simulink model "multiagent"  (R2018b)
settings: Solver=ode4  StartTime=0.0  StopTime=tmax  FixedStep=0.005  RelTol=1e-3
undefined symbols (not defined in the file): dq1_init, dq2_init, dq3_init, dq4_init, q1_init, q2_init, q3_init, q4_init
settings Model: Creator=q5461  LastModifiedBy=q5461

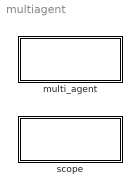
== system multiagent ==
  multi_agent : Subsystem
  scope : Subsystem

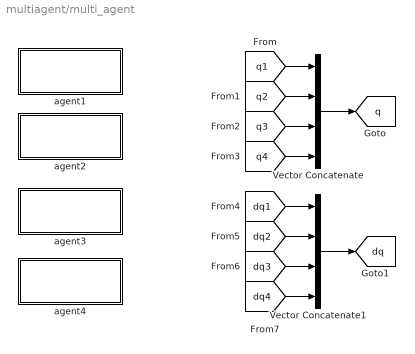
== system multiagent/multi_agent ==
  Vector Concatenate : Concatenate  NumInputs=4
  Vector Concatenate1 : Concatenate  NumInputs=4
  agent1 : Subsystem
  agent2 : Subsystem
  agent3 : Subsystem
  agent4 : Subsystem
  tag scope: dq=global, q=global
  wires:
  [q1] -> Vector Concatenate/1
  [q2] -> Vector Concatenate/2
  Vector Concatenate/1 -> [q]
  [q3] -> Vector Concatenate/3
  [q4] -> Vector Concatenate/4
  [dq4] -> Vector Concatenate1/4
  [dq3] -> Vector Concatenate1/3
  Vector Concatenate1/1 -> [dq]
  [dq2] -> Vector Concatenate1/2
  [dq1] -> Vector Concatenate1/1

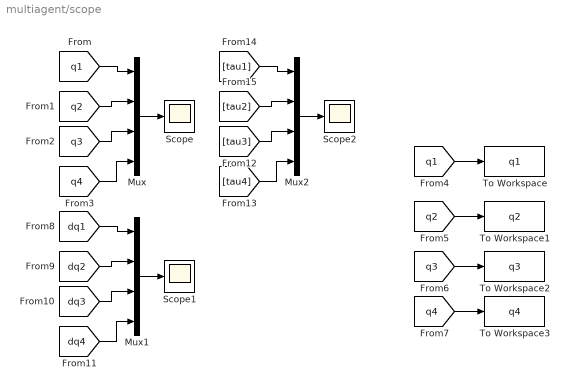
== system multiagent/scope ==
  Mux : Mux
  Mux1 : Mux
  Mux2 : Mux
  Scope : Scope
  Scope1 : Scope
  Scope2 : Scope
  To Workspace : ToWorkspace  VariableName=q1  SaveFormat=Timeseries  SampleTime=-1
  To Workspace1 : ToWorkspace  VariableName=q2  SaveFormat=Timeseries  SampleTime=-1
  To Workspace2 : ToWorkspace  VariableName=q3  SaveFormat=Timeseries  SampleTime=-1
  To Workspace3 : ToWorkspace  VariableName=q4  SaveFormat=Timeseries  SampleTime=-1
  wires:
  Mux/1 -> Scope/1
  [q1] -> Mux/1
  [q2] -> Mux/2
  [q3] -> Mux/3
  [q4] -> Mux/4
  [q1] -> To Workspace/1
  [q2] -> To Workspace1/1
  [q3] -> To Workspace2/1
  [q4] -> To Workspace3/1
  [dq4] -> Mux1/4
  [dq3] -> Mux1/3
  [dq2] -> Mux1/2
  [dq1] -> Mux1/1
  Mux1/1 -> Scope1/1
  Mux2/1 -> Scope2/1
  [tau1] -> Mux2/1
  [tau2] -> Mux2/2
  [tau3] -> Mux2/3
  [tau4] -> Mux2/4

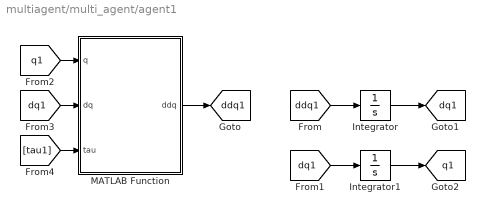
== system multiagent/multi_agent/agent1 ==
  Integrator : Integrator  InitialCondition=dq1_init
  Integrator1 : Integrator  InitialCondition=q1_init
  MATLAB Function : MATLAB Function  TreatAsAtomicUnit=on
  tag scope: ddq1=global, dq1=global, q1=global
  wires:
  [dq1] -> MATLAB Function/2(dq)
  Integrator/1 -> [dq1]
  [dq1] -> Integrator1/1
  Integrator1/1 -> [q1]
  [tau1] -> MATLAB Function/3(tau)
  [q1] -> MATLAB Function/1(q)
  MATLAB Function/1(ddq) -> [ddq1]
  [ddq1] -> Integrator/1

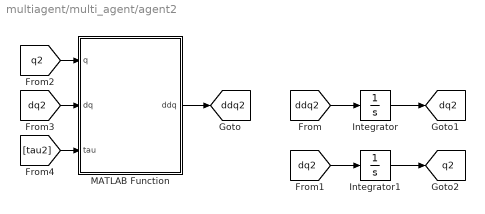
== system multiagent/multi_agent/agent2 ==
  Integrator : Integrator  InitialCondition=dq2_init
  Integrator1 : Integrator  InitialCondition=q2_init
  MATLAB Function : MATLAB Function  TreatAsAtomicUnit=on
  tag scope: ddq2=global, dq2=global, q2=global
  wires:
  [ddq2] -> Integrator/1
  MATLAB Function/1(ddq) -> [ddq2]
  [q2] -> MATLAB Function/1(q)
  [tau2] -> MATLAB Function/3(tau)
  Integrator1/1 -> [q2]
  [dq2] -> Integrator1/1
  Integrator/1 -> [dq2]
  [dq2] -> MATLAB Function/2(dq)

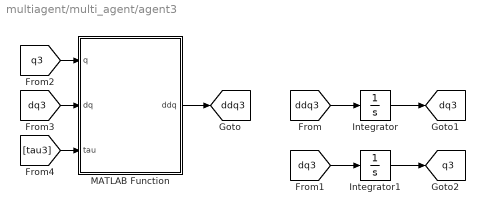
== system multiagent/multi_agent/agent3 ==
  Integrator : Integrator  InitialCondition=dq3_init
  Integrator1 : Integrator  InitialCondition=q3_init
  MATLAB Function : MATLAB Function  TreatAsAtomicUnit=on
  tag scope: ddq3=global, dq3=global, q3=global
  wires:
  [dq3] -> MATLAB Function/2(dq)
  Integrator/1 -> [dq3]
  [dq3] -> Integrator1/1
  Integrator1/1 -> [q3]
  [tau3] -> MATLAB Function/3(tau)
  [q3] -> MATLAB Function/1(q)
  MATLAB Function/1(ddq) -> [ddq3]
  [ddq3] -> Integrator/1

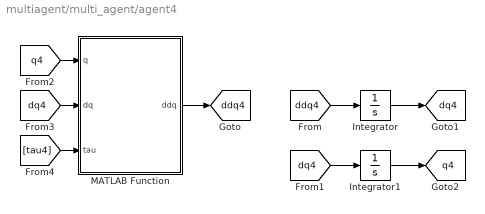
== system multiagent/multi_agent/agent4 ==
  Integrator : Integrator  InitialCondition=dq4_init
  Integrator1 : Integrator  InitialCondition=q4_init
  MATLAB Function : MATLAB Function  TreatAsAtomicUnit=on
  tag scope: ddq4=global, dq4=global, q4=global
  wires:
  [ddq4] -> Integrator/1
  MATLAB Function/1(ddq) -> [ddq4]
  [q4] -> MATLAB Function/1(q)
  [tau4] -> MATLAB Function/3(tau)
  Integrator1/1 -> [q4]
  [dq4] -> Integrator1/1
  Integrator/1 -> [dq4]
  [dq4] -> MATLAB Function/2(dq)

== matlab function multiagent/multi_agent/agent2/MATLAB Function ==
  data: q input; ddq output; dq input; tau input
function ddq = fcn(q,dq,tau)

p1=2.9;p2=0.76;p3=0.87;p4=3.04;p5=0.87;g=9.81;
q1=q(1);q2=q(2);dq1=dq(1);dq2=dq(2);

M=[p1+p2+2*p3*cos(q2) p2+p3*cos(q2);
   p2+p3*cos(q2)      p2];
C=[-p3*dq2*sin(q2) -p3*(dq1+dq2)*sin(q2);
   p3*dq1*sin(q2)  0];
G=[p4*g*cos(q1)+p5*g*cos(q1+q2);p5*g*cos(q1+q2)];

ddq=M\(tau-C*dq-G);

== matlab function multiagent/multi_agent/agent1/MATLAB Function ==
  data: q input; ddq output; dq input; tau input
function ddq = fcn(q,dq,tau)

p1=2.9;p2=0.76;p3=0.87;p4=3.04;p5=0.87;g=9.81;
q1=q(1);q2=q(2);dq1=dq(1);dq2=dq(2);

M=[p1+p2+2*p3*cos(q2) p2+p3*cos(q2);
   p2+p3*cos(q2)      p2];
C=[-p3*dq2*sin(q2) -p3*(dq1+dq2)*sin(q2);
   p3*dq1*sin(q2)  0];
G=[p4*g*cos(q1)+p5*g*cos(q1+q2);p5*g*cos(q1+q2)];

ddq=M\(tau-C*dq-G);

== matlab function multiagent/multi_agent/agent3/MATLAB Function ==
  data: q input; ddq output; dq input; tau input
function ddq = fcn(q,dq,tau)

p1=2.9;p2=0.76;p3=0.87;p4=3.04;p5=0.87;g=9.81;
q1=q(1);q2=q(2);dq1=dq(1);dq2=dq(2);

M=[p1+p2+2*p3*cos(q2) p2+p3*cos(q2);
   p2+p3*cos(q2)      p2];
C=[-p3*dq2*sin(q2) -p3*(dq1+dq2)*sin(q2);
   p3*dq1*sin(q2)  0];
G=[p4*g*cos(q1)+p5*g*cos(q1+q2);p5*g*cos(q1+q2)];

ddq=M\(tau-C*dq-G);

== matlab function multiagent/multi_agent/agent4/MATLAB Function ==
  data: q input; ddq output; dq input; tau input
function ddq = fcn(q,dq,tau)

p1=2.9;p2=0.76;p3=0.87;p4=3.04;p5=0.87;g=9.81;
q1=q(1);q2=q(2);dq1=dq(1);dq2=dq(2);

M=[p1+p2+2*p3*cos(q2) p2+p3*cos(q2);
   p2+p3*cos(q2)      p2];
C=[-p3*dq2*sin(q2) -p3*(dq1+dq2)*sin(q2);
   p3*dq1*sin(q2)  0];
G=[p4*g*cos(q1)+p5*g*cos(q1+q2);p5*g*cos(q1+q2)];

ddq=M\(tau-C*dq-G);
